simulink model "Model"  (R2023b)
settings: Solver=FixedStepAuto  StartTime=0.0  StopTime=10  FixedStep=0.002  RelTol=1e-3
model workspace (MAT data in the model file):
  a = 0
undefined symbols (not defined in the file or in its folder): X, Y, Z
libraries: sm_lib x84, nesl_utility x29, slpidlib x9, simulink x6
(part 4 of 7)

== matlab function Model/支持力结算/MATLAB Function3 ==
  data: m_w input; F_N output; T1 input; T2 input; a_w input; theta input; phi_1 input; phi_4 input; L_0 input
function F_N = fcn(m_w,T1,T2,a_w,theta,phi_1,phi_4,L_0)

l_1=0.15;
l_2=0.27;
l_3=0.27;
l_4=0.15;
l_5=0.15;g=9.80665;

J11=(2*(l_1*cos(phi_1) + (2*l_2*cos(2*atan(((4*l_2^2*(l_1*sin(phi_1) - l_4*sin(phi_4))^2 - ((l_1*sin(phi_1) - l_4*sin(phi_4))^2 + (l_5 - l_1*cos(phi_1) + l_4*cos(phi_4))^2 + l_2^2 - l_3^2)^2 + 4*l_2^2*(l_5 - l_1*cos(phi_1) + l_4*cos(phi_4))^2)^(1/2) - 2*l_2*(l_1*sin(phi_1) - l_4*sin(phi_4)))/((l_1*sin(phi_1) - l_4*sin(phi_4))^2 + (l_5 - l_1*cos(phi_1) + l_4*cos(phi_4))^2 + l_2^2 - l_3^2 + 2*l_2*(l_5 - l_1*cos(phi_1) + l_4*cos(phi_4)))))*(((8*l_1*l_2^2*cos(phi_1)*(l_1*sin(phi_1) - l_4*sin(phi_4)) - 2*(2*l_1*cos(phi_1)*(l_1*sin(phi_1) - l_4*sin(phi_4)) + 2*l_1*sin(phi_1)*(l_5 - l_1*cos(phi_1) + l_4*cos(phi_4)))*((l_1*sin(phi_1) - l_4*sin(phi_4))^2 + (l_5 - l_1*cos(phi_1) + l_4*cos(phi_4))^2 + l_2^2 - l_3^2) + 8*l_1*l_2^2*sin(phi_1)*(l_5 - l_1*cos(phi_1) + l_4*cos(phi_4)))/(2*(4*l_2^2*(l_1*sin(phi_1) - l_4*sin(phi_4))^2 - ((l_1*sin(phi_1) - l_4*sin(phi_4))^2 + (l_5 - l_1*cos(phi_1) + l_4*cos(phi_4))^2 + l_2^2 - l_3^2)^2 + 4*l_2^2*(l_5 - l_1*cos(phi_1) + l_4*cos(phi_4))^2)^(1/2)) - 2*l_1*l_2*cos(phi_1))/((l_1*sin(phi_1) - l_4*sin(phi_4))^2 + (l_5 - l_1*cos(phi_1) + l_4*cos(phi_4))^2 + l_2^2 - l_3^2 + 2*l_2*(l_5 - l_1*cos(phi_1) + l_4*cos(phi_4))) - (((4*l_2^2*(l_1*sin(phi_1) - l_4*sin(phi_4))^2 - ((l_1*sin(phi_1) - l_4*sin(phi_4))^2 + (l_5 - l_1*cos(phi_1) + l_4*cos(phi_4))^2 + l_2^2 - l_3^2)^2 + 4*l_2^2*(l_5 - l_1*cos(phi_1) + l_4*cos(phi_4))^2)^(1/2) - 2*l_2*(l_1*sin(phi_1) - l_4*sin(phi_4)))*(2*l_1*l_2*sin(phi_1) + 2*l_1*cos(phi_1)*(l_1*sin(phi_1) - l_4*sin(phi_4)) + 2*l_1*sin(phi_1)*(l_5 - l_1*cos(phi_1) + l_4*cos(phi_4))))/((l_1*sin(phi_1) - l_4*sin(phi_4))^2 + (l_5 - l_1*cos(phi_1) + l_4*cos(phi_4))^2 + l_2^2 - l_3^2 + 2*l_2*(l_5 - l_1*cos(phi_1) + l_4*cos(phi_4)))^2))/(((4*l_2^2*(l_1*sin(phi_1) - l_4*sin(phi_4))^2 - ((l_1*sin(phi_1) - l_4*sin(phi_4))^2 + (l_5 - l_1*cos(phi_1) + l_4*cos(phi_4))^2 + l_2^2 - l_3^2)^2 + 4*l_2^2*(l_5 - l_1*cos(phi_1) + l_4*cos(phi_4))^2)^(1/2) - 2*l_2*(l_1*sin(phi_1) - l_4*sin(phi_4)))^2/((l_1*sin(phi_1) - l_4*sin(phi_4))^2 + (l_5 - l_1*cos(phi_1) + l_4*cos(phi_4))^2 + l_2^2 - l_3^2 + 2*l_2*(l_5 - l_1*cos(phi_1) + l_4*cos(phi_4)))^2 + 1))*(l_2*sin(2*atan(((4*l_2^2*(l_1*sin(phi_1) - l_4*sin(phi_4))^2 - ((l_1*sin(phi_1) - l_4*sin(phi_4))^2 + (l_5 - l_1*cos(phi_1) + l_4*cos(phi_4))^2 + l_2^2 - l_3^2)^2 + 4*l_2^2*(l_5 - l_1*cos(phi_1) + l_4*cos(phi_4))^2)^(1/2) - 2*l_2*(l_1*sin(phi_1) - l_4*sin(phi_4)))/((l_1*sin(phi_1) - l_4*sin(phi_4))^2 + (l_5 - l_1*cos(phi_1) + l_4*cos(phi_4))^2 + l_2^2 - l_3^2 + 2*l_2*(l_5 - l_1*cos(phi_1) + l_4*cos(phi_4))))) + l_1*sin(phi_1)) - 2*(l_1*sin(phi_1) + (2*l_2*sin(2*atan(((4*l_2^2*(l_1*sin(phi_1) - l_4*sin(phi_4))^2 - ((l_1*sin(phi_1) - l_4*sin(phi_4))^2 + (l_5 - l_1*cos(phi_1) + l_4*cos(phi_4))^2 + l_2^2 - l_3^2)^2 + 4*l_2^2*(l_5 - l_1*cos(phi_1) + l_4*cos(phi_4))^2)^(1/2) - 2*l_2*(l_1*sin(phi_1) - l_4*sin(phi_4)))/((l_1*sin(phi_1) - l_4*sin(phi_4))^2 + (l_5 - l_1*cos(phi_1) + l_4*cos(phi_4))^2 + l_2^2 - l_3^2 + 2*l_2*(l_5 - l_1*cos(phi_1) + l_4*cos(phi_4)))))*(((8*l_1*l_2^2*cos(phi_1)*(l_1*sin(phi_1) - l_4*sin(phi_4)) - 2*(2*l_1*cos(phi_1)*(l_1*sin(phi_1) - l_4*sin(phi_4)) + 2*l_1*sin(phi_1)*(l_5 - l_1*cos(phi_1) + l_4*cos(phi_4)))*((l_1*sin(phi_1) - l_4*sin(phi_4))^2 + (l_5 - l_1*cos(phi_1) + l_4*cos(phi_4))^2 + l_2^2 - l_3^2) + 8*l_1*l_2^2*sin(phi_1)*(l_5 - l_1*cos(phi_1) + l_4*cos(phi_4)))/(2*(4*l_2^2*(l_1*sin(phi_1) - l_4*sin(phi_4))^2 - ((l_1*sin(phi_1) - l_4*sin(phi_4))^2 + (l_5 - l_1*cos(phi_1) + l_4*cos(phi_4))^2 + l_2^2 - l_3^2)^2 + 4*l_2^2*(l_5 - l_1*cos(phi_1) + l_4*cos(phi_4))^2)^(1/2)) - 2*l_1*l_2*cos(phi_1))/((l_1*sin(phi_1) - l_4*sin(phi_4))^2 + (l_5 - l_1*cos(phi_1) + l_4*cos(phi_4))^2 + l_2^2 - l_3^2 + 2*l_2*(l_5 - l_1*cos(phi_1) + l_4*cos(phi_4))) - (((4*l_2^2*(l_1*sin(phi_1) - l_4*sin(phi_4))^2 - ((l_1*sin(phi_1) - l_4*sin(phi_4))^2 + (l_5 - l_1*cos(phi_1) + l_4*cos(phi_4))^2 + l_2^2 - l_3^2)^2 + 4*l_2^2*(l_5 - l_1*cos(phi_1) + l_4*cos(phi_4))^2)^(1/2) - 2*l_2*(l_1*sin(phi_1) - l_4*sin(phi_4)))*(2*l_1*l_2*sin(phi_1) + 2*l_1*cos(phi_1)*(l_1*sin(phi_1) - l_4*sin(phi_4)) + 2*l_1*sin(phi_1)*(l_5 - l_1*cos(phi_1) + l_4*cos(phi_4))))/((l_1*sin(phi_1) - l_4*sin(phi_4))^2 + (l_5 - l_1*cos(phi_1) + l_4*cos(phi_4))^2 + l_2^2 - l_3^2 + 2*l_2*(l_5 - l_1*cos(phi_1) + l_4*cos(phi_4)))^2))/(((4*l_2^2*(l_1*sin(phi_1) - l_4*sin(phi_4))^2 - ((l_1*sin(phi_1) - l_4*sin(phi_4))^2 + (l_5 - l_1*cos(phi_1) + l_4*cos(phi_4))^2 + l_2^2 - l_3^2)^2 + 4*l_2^2*(l_5 - l_1*cos(phi_1) + l_4*cos(phi_4))^2)^(1/2) - 2*l_2*(l_1*sin(phi_1) - l_4*sin(phi_4)))^2/((l_1*sin(phi_1) - l_4*sin(phi_4))^2 + (l_5 - l_1*cos(phi_1) + l_4*cos(phi_4))^2 + l_2^2 - l_3^2 + 2*l_2*(l_5 - l_1*cos(phi_1) + l_4*cos(phi_4)))^2 + 1))*(l_2*cos(2*atan(((4*l_2^2*(l_1*sin(phi_1) - l_4*sin(phi_4))^2 - ((l_1*sin(phi_1) - l_4*sin(phi_4))^2 + (l_5 - l_1*cos(phi_1) + l_4*cos(phi_4))^2 + l_2^2 - l_3^2)^2 + 4*l_2^2*(l_5 - l_1*cos(phi_1) + l_4*cos(phi_4))^2)^(1/2) - 2*l_2*(l_1*sin(phi_1) - l_4*sin(phi_4)))/((l_1*sin(phi_1) - l_4*sin(phi_4))^2 + (l_5 - l_1*cos(phi_1) + l_4*cos(phi_4))^2 + l_2^2 - l_3^2 + 2*l_2*(l_5 - l_1*cos(phi_1) + l_4*cos(phi_4))))) - l_5/2 + l_1*cos(phi_1)))/(2*((l_2*sin(2*atan(((4*l_2^2*(l_1*sin(phi_1) - l_4*sin(phi_4))^2 - ((l_1*sin(phi_1) - l_4*sin(phi_4))^2 + (l_5 - l_1*cos(phi_1) + l_4*cos(phi_4))^2 + l_2^2 - l_3^2)^2 + 4*l_2^2*(l_5 - l_1*cos(phi_1) + l_4*cos(phi_4))^2)^(1/2) - 2*l_2*(l_1*sin(phi_1) - l_4*sin(phi_4)))/((l_1*sin(phi_1) - l_4*sin(phi_4))^2 + (l_5 - l_1*cos(phi_1) + l_4*cos(phi_4))^2 + l_2^2 - l_3^2 + 2*l_2*(l_5 - l_1*cos(phi_1) + l_4*cos(phi_4))))) + l_1*sin(phi_1))^2 + (l_2*cos(2*atan(((4*l_2^2*(l_1*sin(phi_1) - l_4*sin(phi_4))^2 - ((l_1*sin(phi_1) - l_4*sin(phi_4))^2 + (l_5 - l_1*cos(phi_1) + l_4*cos(phi_4))^2 + l_2^2 - l_3^2)^2 + 4*l_2^2*(l_5 - l_1*cos(phi_1) + l_4*cos(phi_4))^2)^(1/2) - 2*l_2*(l_1*sin(phi_1) - l_4*sin(phi_4)))/((l_1*sin(phi_1) - l_4*sin(phi_4))^2 + (l_5 - l_1*cos(phi_1) + l_4*cos(phi_4))^2 + l_2^2 - l_3^2 + 2*l_2*(l_5 - l_1*cos(phi_1) + l_4*cos(phi_4))))) - l_5/2 + l_1*cos(phi_1))^2)^(1/2));
J12=((4*l_2*sin(2*atan(((4*l_2^2*(l_1*sin(phi_1) - l_4*sin(phi_4))^2 - ((l_1*sin(phi_1) - l_4*sin(phi_4))^2 + (l_5 - l_1*cos(phi_1) + l_4*cos(phi_4))^2 + l_2^2 - l_3^2)^2 + 4*l_2^2*(l_5 - l_1*cos(phi_1) + l_4*cos(phi_4))^2)^(1/2) - 2*l_2*(l_1*sin(phi_1) - l_4*sin(phi_4)))/((l_1*sin(phi_1) - l_4*sin(phi_4))^2 + (l_5 - l_1*cos(phi_1) + l_4*cos(phi_4))^2 + l_2^2 - l_3^2 + 2*l_2*(l_5 - l_1*cos(phi_1) + l_4*cos(phi_4)))))*(((8*l_2^2*l_4*cos(phi_4)*(l_1*sin(phi_1) - l_4*sin(phi_4)) - 2*(2*l_4*cos(phi_4)*(l_1*sin(phi_1) - l_4*sin(phi_4)) + 2*l_4*sin(phi_4)*(l_5 - l_1*cos(phi_1) + l_4*cos(phi_4)))*((l_1*sin(phi_1) - l_4*sin(phi_4))^2 + (l_5 - l_1*cos(phi_1) + l_4*cos(phi_4))^2 + l_2^2 - l_3^2) + 8*l_2^2*l_4*sin(phi_4)*(l_5 - l_1*cos(phi_1) + l_4*cos(phi_4)))/(2*(4*l_2^2*(l_1*sin(phi_1) - l_4*sin(phi_4))^2 - ((l_1*sin(phi_1) - l_4*sin(phi_4))^2 + (l_5 - l_1*cos(phi_1) + l_4*cos(phi_4))^2 + l_2^2 - l_3^2)^2 + 4*l_2^2*(l_5 - l_1*cos(phi_1) + l_4*cos(phi_4))^2)^(1/2)) - 2*l_2*l_4*cos(phi_4))/((l_1*sin(phi_1) - l_4*sin(phi_4))^2 + (l_5 - l_1*cos(phi_1) + l_4*cos(phi_4))^2 + l_2^2 - l_3^2 + 2*l_2*(l_5 - l_1*cos(phi_1) + l_4*cos(phi_4))) - (((4*l_2^2*(l_1*sin(phi_1) - l_4*sin(phi_4))^2 - ((l_1*sin(phi_1) - l_4*sin(phi_4))^2 + (l_5 - l_1*cos(phi_1) + l_4*cos(phi_4))^2 + l_2^2 - l_3^2)^2 + 4*l_2^2*(l_5 - l_1*cos(phi_1) + l_4*cos(phi_4))^2)^(1/2) - 2*l_2*(l_1*sin(phi_1) - l_4*sin(phi_4)))*(2*l_2*l_4*sin(phi_4) + 2*l_4*cos(phi_4)*(l_1*sin(phi_1) - l_4*sin(phi_4)) + 2*l_4*sin(phi_4)*(l_5 - l_1*cos(phi_1) + l_4*cos(phi_4))))/((l_1*sin(phi_1) - l_4*sin(phi_4))^2 + (l_5 - l_1*cos(phi_1) + l_4*cos(phi_4))^2 + l_2^2 - l_3^2 + 2*l_2*(l_5 - l_1*cos(phi_1) + l_4*cos(phi_4)))^2)*(l_2*cos(2*atan(((4*l_2^2*(l_1*sin(phi_1) - l_4*sin(phi_4))^2 - ((l_1*sin(phi_1) - l_4*sin(phi_4))^2 + (l_5 - l_1*cos(phi_1) + l_4*cos(phi_4))^2 + l_2^2 - l_3^2)^2 + 4*l_2^2*(l_5 - l_1*cos(phi_1) + l_4*cos(phi_4))^2)^(1/2) - 2*l_2*(l_1*sin(phi_1) - l_4*sin(phi_4)))/((l_1*sin(phi_1) - l_4*sin(phi_4))^2 + (l_5 - l_1*cos(phi_1) + l_4*cos(phi_4))^2 + l_2^2 - l_3^2 + 2*l_2*(l_5 - l_1*cos(phi_1) + l_4*cos(phi_4))))) - l_5/2 + l_1*cos(phi_1)))/(((4*l_2^2*(l_1*sin(phi_1) - l_4*sin(phi_4))^2 - ((l_1*sin(phi_1) - l_4*sin(phi_4))^2 + (l_5 - l_1*cos(phi_1) + l_4*cos(phi_4))^2 + l_2^2 - l_3^2)^2 + 4*l_2^2*(l_5 - l_1*cos(phi_1) + l_4*cos(phi_4))^2)^(1/2) - 2*l_2*(l_1*sin(phi_1) - l_4*sin(phi_4)))^2/((l_1*sin(phi_1) - l_4*sin(phi_4))^2 + (l_5 - l_1*cos(phi_1) + l_4*cos(phi_4))^2 + l_2^2 - l_3^2 + 2*l_2*(l_5 - l_1*cos(phi_1) + l_4*cos(phi_4)))^2 + 1) - (4*l_2*cos(2*atan(((4*l_2^2*(l_1*sin(phi_1) - l_4*sin(phi_4))^2 - ((l_1*sin(phi_1) - l_4*sin(phi_4))^2 + (l_5 - l_1*cos(phi_1) + l_4*cos(phi_4))^2 + l_2^2 - l_3^2)^2 + 4*l_2^2*(l_5 - l_1*cos(phi_1) + l_4*cos(phi_4))^2)^(1/2) - 2*l_2*(l_1*sin(phi_1) - l_4*sin(phi_4)))/((l_1*sin(phi_1) - l_4*sin(phi_4))^2 + (l_5 - l_1*cos(phi_1) + l_4*cos(phi_4))^2 + l_2^2 - l_3^2 + 2*l_2*(l_5 - l_1*cos(phi_1) + l_4*cos(phi_4)))))*(l_2*sin(2*atan(((4*l_2^2*(l_1*sin(phi_1) - l_4*sin(phi_4))^2 - ((l_1*sin(phi_1) - l_4*sin(phi_4))^2 + (l_5 - l_1*cos(phi_1) + l_4*cos(phi_4))^2 + l_2^2 - l_3^2)^2 + 4*l_2^2*(l_5 - l_1*cos(phi_1) + l_4*cos(phi_4))^2)^(1/2) - 2*l_2*(l_1*sin(phi_1) - l_4*sin(phi_4)))/((l_1*sin(phi_1) - l_4*sin(phi_4))^2 + (l_5 - l_1*cos(phi_1) + l_4*cos(phi_4))^2 + l_2^2 - l_3^2 + 2*l_2*(l_5 - l_1*cos(phi_1) + l_4*cos(phi_4))))) + l_1*sin(phi_1))*(((8*l_2^2*l_4*cos(phi_4)*(l_1*sin(phi_1) - l_4*sin(phi_4)) - 2*(2*l_4*cos(phi_4)*(l_1*sin(phi_1) - l_4*sin(phi_4)) + 2*l_4*sin(phi_4)*(l_5 - l_1*cos(phi_1) + l_4*cos(phi_4)))*((l_1*sin(phi_1) - l_4*sin(phi_4))^2 + (l_5 - l_1*cos(phi_1) + l_4*cos(phi_4))^2 + l_2^2 - l_3^2) + 8*l_2^2*l_4*sin(phi_4)*(l_5 - l_1*cos(phi_1) + l_4*cos(phi_4)))/(2*(4*l_2^2*(l_1*sin(phi_1) - l_4*sin(phi_4))^2 - ((l_1*sin(phi_1) - l_4*sin(phi_4))^2 + (l_5 - l_1*cos(phi_1) + l_4*cos(phi_4))^2 + l_2^2 - l_3^2)^2 + 4*l_2^2*(l_5 - l_1*cos(phi_1) + l_4*cos(phi_4))^2)^(1/2)) - 2*l_2*l_4*cos(phi_4))/((l_1*sin(phi_1) - l_4*sin(phi_4))^2 + (l_5 - l_1*cos(phi_1) + l_4*cos(phi_4))^2 + l_2^2 - l_3^2 + 2*l_2*(l_5 - l_1*cos(phi_1) + l_4*cos(phi_4))) - (((4*l_2^2*(l_1*sin(phi_1) - l_4*sin(phi_4))^2 - ((l_1*sin(phi_1) - l_4*sin(phi_4))^2 + (l_5 - l_1*cos(phi_1) + l_4*cos(phi_4))^2 + l_2^2 - l_3^2)^2 + 4*l_2^2*(l_5 - l_1*cos(phi_1) + l_4*cos(phi_4))^2)^(1/2) - 2*l_2*(l_1*sin(phi_1) - l_4*sin(phi_4)))*(2*l_2*l_4*sin(phi_4) + 2*l_4*cos(phi_4)*(l_1*sin(phi_1) - l_4*sin(phi_4)) + 2*l_4*sin(phi_4)*(l_5 - l_1*cos(phi_1) + l_4*cos(phi_4))))/((l_1*sin(phi_1) - l_4*sin(phi_4))^2 + (l_5 - l_1*cos(phi_1) + l_4*cos(phi_4))^2 + l_2^2 - l_3^2 + 2*l_2*(l_5 - l_1*cos(phi_1) + l_4*cos(phi_4)))^2))/(((4*l_2^2*(l_1*sin(phi_1) - l_4*sin(phi_4))^2 - ((l_1*sin(phi_1) - l_4*sin(phi_4))^2 + (l_5 - l_1*cos(phi_1) + l_4*cos(phi_4))^2 + l_2^2 - l_3^2)^2 + 4*l_2^2*(l_5 - l_1*cos(phi_1) + l_4*cos(phi_4))^2)^(1/2) - 2*l_2*(l_1*sin(phi_1) - l_4*sin(phi_4)))^2/((l_1*sin(phi_1) - l_4*sin(phi_4))^2 + (l_5 - l_1*cos(phi_1) + l_4*cos(phi_4))^2 + l_2^2 - l_3^2 + 2*l_2*(l_5 - l_1*cos(phi_1) + l_4*cos(phi_4)))^2 + 1))/(2*((l_2*sin(2*atan(((4*l_2^2*(l_1*sin(phi_1) - l_4*sin(phi_4))^2 - ((l_1*sin(phi_1) - l_4*sin(phi_4))^2 + (l_5 - l_1*cos(phi_1) + l_4*cos(phi_4))^2 + l_2^2 - l_3^2)^2 + 4*l_2^2*(l_5 - l_1*cos(phi_1) + l_4*cos(phi_4))^2)^(1/2) - 2*l_2*(l_1*sin(phi_1) - l_4*sin(phi_4)))/((l_1*sin(phi_1) - l_4*sin(phi_4))^2 + (l_5 - l_1*cos(phi_1) + l_4*cos(phi_4))^2 + l_2^2 - l_3^2 + 2*l_2*(l_5 - l_1*cos(phi_1) + l_4*cos(phi_4))))) + l_1*sin(phi_1))^2 + (l_2*cos(2*atan(((4*l_2^2*(l_1*sin(phi_1) - l_4*sin(phi_4))^2 - ((l_1*sin(phi_1) - l_4*sin(phi_4))^2 + (l_5 - l_1*cos(phi_1) + l_4*cos(phi_4))^2 + l_2^2 - l_3^2)^2 + 4*l_2^2*(l_5 - l_1*cos(phi_1) + l_4*cos(phi_4))^2)^(1/2) - 2*l_2*(l_1*sin(phi_1) - l_4*sin(phi_4)))/((l_1*sin(phi_1) - l_4*sin(phi_4))^2 + (l_5 - l_1*cos(phi_1) + l_4*cos(phi_4))^2 + l_2^2 - l_3^2 + 2*l_2*(l_5 - l_1*cos(phi_1) + l_4*cos(phi_4))))) - l_5/2 + l_1*cos(phi_1))^2)^(1/2));
J21=((l_1*sin(phi_1) + (2*l_2*sin(2*atan(((4*l_2^2*(l_1*sin(phi_1) - l_4*sin(phi_4))^2 - ((l_1*sin(phi_1) - l_4*sin(phi_4))^2 + (l_5 - l_1*cos(phi_1) + l_4*cos(phi_4))^2 + l_2^2 - l_3^2)^2 + 4*l_2^2*(l_5 - l_1*cos(phi_1) + l_4*cos(phi_4))^2)^(1/2) - 2*l_2*(l_1*sin(phi_1) - l_4*sin(phi_4)))/((l_1*sin(phi_1) - l_4*sin(phi_4))^2 + (l_5 - l_1*cos(phi_1) + l_4*cos(phi_4))^2 + l_2^2 - l_3^2 + 2*l_2*(l_5 - l_1*cos(phi_1) + l_4*cos(phi_4)))))*(((8*l_1*l_2^2*cos(phi_1)*(l_1*sin(phi_1) - l_4*sin(phi_4)) - 2*(2*l_1*cos(phi_1)*(l_1*sin(phi_1) - l_4*sin(phi_4)) + 2*l_1*sin(phi_1)*(l_5 - l_1*cos(phi_1) + l_4*cos(phi_4)))*((l_1*sin(phi_1) - l_4*sin(phi_4))^2 + (l_5 - l_1*cos(phi_1) + l_4*cos(phi_4))^2 + l_2^2 - l_3^2) + 8*l_1*l_2^2*sin(phi_1)*(l_5 - l_1*cos(phi_1) + l_4*cos(phi_4)))/(2*(4*l_2^2*(l_1*sin(phi_1) - l_4*sin(phi_4))^2 - ((l_1*sin(phi_1) - l_4*sin(phi_4))^2 + (l_5 - l_1*cos(phi_1) + l_4*cos(phi_4))^2 + l_2^2 - l_3^2)^2 + 4*l_2^2*(l_5 - l_1*cos(phi_1) + l_4*cos(phi_4))^2)^(1/2)) - 2*l_1*l_2*cos(phi_1))/((l_1*sin(phi_1) - l_4*sin(phi_4))^2 + (l_5 - l_1*cos(phi_1) + l_4*cos(phi_4))^2 + l_2^2 - l_3^2 + 2*l_2*(l_5 - l_1*cos(phi_1) + l_4*cos(phi_4))) - (((4*l_2^2*(l_1*sin(phi_1) - l_4*sin(phi_4))^2 - ((l_1*sin(phi_1) - l_4*sin(phi_4))^2 + (l_5 - l_1*cos(phi_1) + l_4*cos(phi_4))^2 + l_2^2 - l_3^2)^2 + 4*l_2^2*(l_5 - l_1*cos(phi_1) + l_4*cos(phi_4))^2)^(1/2) - 2*l_2*(l_1*sin(phi_1) - l_4*sin(phi_4)))*(2*l_1*l_2*sin(phi_1) + 2*l_1*cos(phi_1)*(l_1*sin(phi_1) - l_4*sin(phi_4)) + 2*l_1*sin(phi_1)*(l_5 - l_1*cos(phi_1) + l_4*cos(phi_4))))/((l_1*sin(phi_1) - l_4*sin(phi_4))^2 + (l_5 - l_1*cos(phi_1) + l_4*cos(phi_4))^2 + l_2^2 - l_3^2 + 2*l_2*(l_5 - l_1*cos(phi_1) + l_4*cos(phi_4)))^2))/(((4*l_2^2*(l_1*sin(phi_1) - l_4*sin(phi_4))^2 - ((l_1*sin(phi_1) - l_4*sin(phi_4))^2 + (l_5 - l_1*cos(phi_1) + l_4*cos(phi_4))^2 + l_2^2 - l_3^2)^2 + 4*l_2^2*(l_5 - l_1*cos(phi_1) + l_4*cos(phi_4))^2)^(1/2) - 2*l_2*(l_1*sin(phi_1) - l_4*sin(phi_4)))^2/((l_1*sin(phi_1) - l_4*sin(phi_4))^2 + (l_5 - l_1*cos(phi_1) + l_4*cos(phi_4))^2 + l_2^2 - l_3^2 + 2*l_2*(l_5 - l_1*cos(phi_1) + l_4*cos(phi_4)))^2 + 1))/((l_2*sin(2*atan(((4*l_2^2*(l_1*sin(phi_1) - l_4*sin(phi_4))^2 - ((l_1*sin(phi_1) - l_4*sin(phi_4))^2 + (l_5 - l_1*cos(phi_1) + l_4*cos(phi_4))^2 + l_2^2 - l_3^2)^2 + 4*l_2^2*(l_5 - l_1*cos(phi_1) + l_4*cos(phi_4))^2)^(1/2) - 2*l_2*(l_1*sin(phi_1) - l_4*sin(phi_4)))/((l_1*sin(phi_1) - l_4*sin(phi_4))^2 + (l_5 - l_1*cos(phi_1) + l_4*cos(phi_4))^2 + l_2^2 - l_3^2 + 2*l_2*(l_5 - l_1*cos(phi_1) + l_4*cos(phi_4))))) + l_1*sin(phi_1))^2 + (l_2*cos(2*atan(((4*l_2^2*(l_1*sin(phi_1) - l_4*sin(phi_4))^2 - ((l_1*sin(phi_1) - l_4*sin(phi_4))^2 + (l_5 - l_1*cos(phi_1) + l_4*cos(phi_4))^2 + l_2^2 - l_3^2)^2 + 4*l_2^2*(l_5 - l_1*cos(phi_1) + l_4*cos(phi_4))^2)^(1/2) - 2*l_2*(l_1*sin(phi_1) - l_4*sin(phi_4)))/((l_1*sin(phi_1) - l_4*sin(phi_4))^2 + (l_5 - l_1*cos(phi_1) + l_4*cos(phi_4))^2 + l_2^2 - l_3^2 + 2*l_2*(l_5 - l_1*cos(phi_1) + l_4*cos(phi_4))))) - l_5/2 + l_1*cos(phi_1))^2)^(1/2) + ((2*(l_1*cos(phi_1) + (2*l_2*cos(2*atan(((4*l_2^2*(l_1*sin(phi_1) - l_4*sin(phi_4))^2 - ((l_1*sin(phi_1) - l_4*sin(phi_4))^2 + (l_5 - l_1*cos(phi_1) + l_4*cos(phi_4))^2 + l_2^2 - l_3^2)^2 + 4*l_2^2*(l_5 - l_1*cos(phi_1) + l_4*cos(phi_4))^2)^(1/2) - 2*l_2*(l_1*sin(phi_1) - l_4*sin(phi_4)))/((l_1*sin(phi_1) - l_4*sin(phi_4))^2 + (l_5 - l_1*cos(phi_1) + l_4*cos(phi_4))^2 + l_2^2 - l_3^2 + 2*l_2*(l_5 - l_1*cos(phi_1) + l_4*cos(phi_4)))))*(((8*l_1*l_2^2*cos(phi_1)*(l_1*sin(phi_1) - l_4*sin(phi_4)) - 2*(2*l_1*cos(phi_1)*(l_1*sin(phi_1) - l_4*sin(phi_4)) + 2*l_1*sin(phi_1)*(l_5 - l_1*cos(phi_1) + l_4*cos(phi_4)))*((l_1*sin(phi_1) - l_4*sin(phi_4))^2 + (l_5 - l_1*cos(phi_1) + l_4*cos(phi_4))^2 + l_2^2 - l_3^2) + 8*l_1*l_2^2*sin(phi_1)*(l_5 - l_1*cos(phi_1) + l_4*cos(phi_4)))/(2*(4*l_2^2*(l_1*sin(phi_1) - l_4*sin(phi_4))^2 - ((l_1*sin(phi_1) - l_4*sin(phi_4))^2 + (l_5 - l_1*cos(phi_1) + l_4*cos(phi_4))^2 + l_2^2 - l_3^2)^2 + 4*l_2^2*(l_5 - l_1*cos(phi_1) + l_4*cos(phi_4))^2)^(1/2)) - 2*l_1*l_2*cos(phi_1))/((l_1*sin(phi_1) - l_4*sin(phi_4))^2 + (l_5 - l_1*cos(phi_1) + l_4*cos(phi_4))^2 + l_2^2 - l_3^2 + 2*l_2*(l_5 - l_1*cos(phi_1) + l_4*cos(phi_4))) - (((4*l_2^2*(l_1*sin(phi_1) - l_4*sin(phi_4))^2 - ((l_1*sin(phi_1) - l_4*sin(phi_4))^2 + (l_5 - l_1*cos(phi_1) + l_4*cos(phi_4))^2 + l_2^2 - l_3^2)^2 + 4*l_2^2*(l_5 - l_1*cos(phi_1) + l_4*cos(phi_4))^2)^(1/2) - 2*l_2*(l_1*sin(phi_1) - l_4*sin(phi_4)))*(2*l_1*l_2*sin(phi_1) + 2*l_1*cos(phi_1)*(l_1*sin(phi_1) - l_4*sin(phi_4)) + 2*l_1*sin(phi_1)*(l_5 - l_1*cos(phi_1) + l_4*cos(phi_4))))/((l_1*sin(phi_1) - l_4*sin(phi_4))^2 + (l_5 - l_1*cos(phi_1) + l_4*cos(phi_4))^2 + l_2^2 - l_3^2 + 2*l_2*(l_5 - l_1*cos(phi_1) + l_4*cos(phi_4)))^2))/(((4*l_2^2*(l_1*sin(phi_1) - l_4*sin(phi_4))^2 - ((l_1*sin(phi_1) - l_4*sin(phi_4))^2 + (l_5 - l_1*cos(phi_1) + l_4*cos(phi_4))^2 + l_2^2 - l_3^2)^2 + 4*l_2^2*(l_5 - l_1*cos(phi_1) + l_4*cos(phi_4))^2)^(1/2) - 2*l_2*(l_1*sin(phi_1) - l_4*sin(phi_4)))^2/((l_1*sin(phi_1) - l_4*sin(phi_4))^2 + (l_5 - l_1*cos(phi_1) + l_4*cos(phi_4))^2 + l_2^2 - l_3^2 + 2*l_2*(l_5 - l_1*cos(phi_1) + l_4*cos(phi_4)))^2 + 1))*(l_2*sin(2*atan(((4*l_2^2*(l_1*sin(phi_1) - l_4*sin(phi_4))^2 - ((l_1*sin(phi_1) - l_4*sin(phi_4))^2 + (l_5 - l_1*cos(phi_1) + l_4*cos(phi_4))^2 + l_2^2 - l_3^2)^2 + 4*l_2^2*(l_5 - l_1*cos(phi_1) + l_4*cos(phi_4))^2)^(1/2) - 2*l_2*(l_1*sin(phi_1) - l_4*sin(phi_4)))/((l_1*sin(phi_1) - l_4*sin(phi_4))^2 + (l_5 - l_1*cos(phi_1) + l_4*cos(phi_4))^2 + l_2^2 - l_3^2 + 2*l_2*(l_5 - l_1*cos(phi_1) + l_4*cos(phi_4))))) + l_1*sin(phi_1)) - 2*(l_1*sin(phi_1) + (2*l_2*sin(2*atan(((4*l_2^2*(l_1*sin(phi_1) - l_4*sin(phi_4))^2 - ((l_1*sin(phi_1) - l_4*sin(phi_4))^2 + (l_5 - l_1*cos(phi_1) + l_4*cos(phi_4))^2 + l_2^2 - l_3^2)^2 + 4*l_2^2*(l_5 - l_1*cos(phi_1) + l_4*cos(phi_4))^2)^(1/2) - 2*l_2*(l_1*sin(phi_1) - l_4*sin(phi_4)))/((l_1*sin(phi_1) - l_4*sin(phi_4))^2 + (l_5 - l_1*cos(phi_1) + l_4*cos(phi_4))^2 + l_2^2 - l_3^2 + 2*l_2*(l_5 - l_1*cos(phi_1) + l_4*cos(phi_4)))))*(((8*l_1*l_2^2*cos(phi_1)*(l_1*sin(phi_1) - l_4*sin(phi_4)) - 2*(2*l_1*cos(phi_1)*(l_1*sin(phi_1) - l_4*sin(phi_4)) + 2*l_1*sin(phi_1)*(l_5 - l_1*cos(phi_1) + l_4*cos(phi_4)))*((l_1*sin(phi_1) - l_4*sin(phi_4))^2 + (l_5 - l_1*cos(phi_1) + l_4*cos(phi_4))^2 + l_2^2 - l_3^2) + 8*l_1*l_2^2*sin(phi_1)*(l_5 - l_1*cos(phi_1) + l_4*cos(phi_4)))/(2*(4*l_2^2*(l_1*sin(phi_1) - l_4*sin(phi_4))^2 - ((l_1*sin(phi_1) - l_4*sin(phi_4))^2 + (l_5 - l_1*cos(phi_1) + l_4*cos(phi_4))^2 + l_2^2 - l_3^2)^2 + 4*l_2^2*(l_5 - l_1*cos(phi_1) + l_4*cos(phi_4))^2)^(1/2)) - 2*l_1*l_2*cos(phi_1))/((l_1*sin(phi_1) - l_4*sin(phi_4))^2 + (l_5 - l_1*cos(phi_1) + l_4*cos(phi_4))^2 + l_2^2 - l_3^2 + 2*l_2*(l_5 - l_1*cos(phi_1) + l_4*cos(phi_4))) - (((4*l_2^2*(l_1*sin(phi_1) - l_4*sin(phi_4))^2 - ((l_1*sin(phi_1) - l_4*sin(phi_4))^2 + (l_5 - l_1*cos(phi_1) + l_4*cos(phi_4))^2 + l_2^2 - l_3^2)^2 + 4*l_2^2*(l_5 - l_1*cos(phi_1) + l_4*cos(phi_4))^2)^(1/2) - 2*l_2*(l_1*sin(phi_1) - l_4*sin(phi_4)))*(2*l_1*l_2*sin(phi_1) + 2*l_1*cos(phi_1)*(l_1*sin(phi_1) - l_4*sin(phi_4)) + 2*l_1*sin(phi_1)*(l_5 - l_1*cos(phi_1) + l_4*cos(phi_4))))/((l_1*sin(phi_1) - l_4*sin(phi_4))^2 + (l_5 - l_1*cos(phi_1) + l_4*cos(phi_4))^2 + l_2^2 - l_3^2 + 2*l_2*(l_5 - l_1*cos(phi_1) + l_4*cos(phi_4)))^2))/(((4*l_2^2*(l_1*sin(phi_1) - l_4*sin(phi_4))^2 - ((l_1*sin(phi_1) - l_4*sin(phi_4))^2 + (l_5 - l_1*cos(phi_1) + l_4*cos(phi_4))^2 + l_2^2 - l_3^2)^2 + 4*l_2^2*(l_5 - l_1*cos(phi_1) + l_4*cos(phi_4))^2)^(1/2) - 2*l_2*(l_1*sin(phi_1) - l_4*sin(phi_4)))^2/((l_1*sin(phi_1) - l_4*sin(phi_4))^2 + (l_5 - l_1*cos(phi_1) + l_4*cos(phi_4))^2 + l_2^2 - l_3^2 + 2*l_2*(l_5 - l_1*cos(phi_1) + l_4*cos(phi_4)))^2 + 1))*(l_2*cos(2*atan(((4*l_2^2*(l_1*sin(phi_1) - l_4*sin(phi_4))^2 - ((l_1*sin(phi_1) - l_4*sin(phi_4))^2 + (l_5 - l_1*cos(phi_1) + l_4*cos(phi_4))^2 + l_2^2 - l_3^2)^2 + 4*l_2^2*(l_5 - l_1*cos(phi_1) + l_4*cos(phi_4))^2)^(1/2) - 2*l_2*(l_1*sin(phi_1) - l_4*sin(phi_4)))/((l_1*sin(phi_1) - l_4*sin(phi_4))^2 + (l_5 - l_1*cos(phi_1) + l_4*cos(phi_4))^2 + l_2^2 - l_3^2 + 2*l_2*(l_5 - l_1*cos(phi_1) + l_4*cos(phi_4))))) - l_5/2 + l_1*cos(phi_1)))*(l_2*cos(2*atan(((4*l_2^2*(l_1*sin(phi_1) - l_4*sin(phi_4))^2 - ((l_1*sin(phi_1) - l_4*sin(phi_4))^2 + (l_5 - l_1*cos(phi_1) + l_4*cos(phi_4))^2 + l_2^2 - l_3^2)^2 + 4*l_2^2*(l_5 - l_1*cos(phi_1) + l_4*cos(phi_4))^2)^(1/2) - 2*l_2*(l_1*sin(phi_1) - l_4*sin(phi_4)))/((l_1*sin(phi_1) - l_4*sin(phi_4))^2 + (l_5 - l_1*cos(phi_1) + l_4*cos(phi_4))^2 + l_2^2 - l_3^2 + 2*l_2*(l_5 - l_1*cos(phi_1) + l_4*cos(phi_4))))) - l_5/2 + l_1*cos(phi_1)))/(2*((l_2*sin(2*atan(((4*l_2^2*(l_1*sin(phi_1) - l_4*sin(phi_4))^2 - ((l_1*sin(phi_1) - l_4*sin(phi_4))^2 + (l_5 - l_1*cos(phi_1) + l_4*cos(phi_4))^2 + l_2^2 - l_3^2)^2 + 4*l_2^2*(l_5 - l_1*cos(phi_1) + l_4*cos(phi_4))^2)^(1/2) - 2*l_2*(l_1*sin(phi_1) - l_4*sin(phi_4)))/((l_1*sin(phi_1) - l_4*sin(phi_4))^2 + (l_5 - l_1*cos(phi_1) + l_4*cos(phi_4))^2 + l_2^2 - l_3^2 + 2*l_2*(l_5 - l_1*cos(phi_1) + l_4*cos(phi_4))))) + l_1*sin(phi_1))^2 + (l_2*cos(2*atan(((4*l_2^2*(l_1*sin(phi_1) - l_4*sin(phi_4))^2 - ((l_1*sin(phi_1) - l_4*sin(phi_4))^2 + (l_5 - l_1*cos(phi_1) + l_4*cos(phi_4))^2 + l_2^2 - l_3^2)^2 + 4*l_2^2*(l_5 - l_1*cos(phi_1) + l_4*cos(phi_4))^2)^(1/2) - 2*l_2*(l_1*sin(phi_1) - l_4*sin(phi_4)))/((l_1*sin(phi_1) - l_4*sin(phi_4))^2 + (l_5 - l_1*cos(phi_1) + l_4*cos(phi_4))^2 + l_2^2 - l_3^2 + 2*l_2*(l_5 - l_1*cos(phi_1) + l_4*cos(phi_4))))) - l_5/2 + l_1*cos(phi_1))^2)^(3/2)))/(1 - (l_2*cos(2*atan(((4*l_2^2*(l_1*sin(phi_1) - l_4*sin(phi_4))^2 - ((l_1*sin(phi_1) - l_4*sin(phi_4))^2 + (l_5 - l_1*cos(phi_1) + l_4*cos(phi_4))^2 + l_2^2 - l_3^2)^2 + 4*l_2^2*(l_5 - l_1*cos(phi_1) + l_4*cos(phi_4))^2)^(1/2) - 2*l_2*(l_1*sin(phi_1) - l_4*sin(phi_4)))/((l_1*sin(phi_1) - l_4*sin(phi_4))^2 + (l_5 - l_1*cos(phi_1) + l_4*cos(phi_4))^2 + l_2^2 - l_3^2 + 2*l_2*(l_5 - l_1*cos(phi_1) + l_4*cos(phi_4))))) - l_5/2 + l_1*cos(phi_1))^2/((l_2*sin(2*atan(((4*l_2^2*(l_1*sin(phi_1) - l_4*sin(phi_4))^2 - ((l_1*sin(phi_1) - l_4*sin(phi_4))^2 + (l_5 - l_1*cos(phi_1) + l_4*cos(phi_4))^2 + l_2^2 - l_3^2)^2 + 4*l_2^2*(l_5 - l_1*cos(phi_1) + l_4*cos(phi_4))^2)^(1/2) - 2*l_2*(l_1*sin(phi_1) - l_4*sin(phi_4)))/((l_1*sin(phi_1) - l_4*sin(phi_4))^2 + (l_5 - l_1*cos(phi_1) + l_4*cos(phi_4))^2 + l_2^2 - l_3^2 + 2*l_2*(l_5 - l_1*cos(phi_1) + l_4*cos(phi_4))))) + l_1*sin(phi_1))^2 + (l_2*cos(2*atan(((4*l_2^2*(l_1*sin(phi_1) - l_4*sin(phi_4))^2 - ((l_1*sin(phi_1) - l_4*sin(phi_4))^2 + (l_5 - l_1*cos(phi_1) + l_4*cos(phi_4))^2 + l_2^2 - l_3^2)^2 + 4*l_2^2*(l_5 - l_1*cos(phi_1) + l_4*cos(phi_4))^2)^(1/2) - 2*l_2*(l_1*sin(phi_1) - l_4*sin(phi_4)))/((l_1*sin(phi_1) - l_4*sin(phi_4))^2 + (l_5 - l_1*cos(phi_1) + l_4*cos(phi_4))^2 + l_2^2 - l_3^2 + 2*l_2*(l_5 - l_1*cos(phi_1) + l_4*cos(phi_4))))) - l_5/2 + l_1*cos(phi_1))^2))^(1/2);
J22=((((4*l_2*sin(2*atan(((4*l_2^2*(l_1*sin(phi_1) - l_4*sin(phi_4))^2 - ((l_1*sin(phi_1) - l_4*sin(phi_4))^2 + (l_5 - l_1*cos(phi_1) + l_4*cos(phi_4))^2 + l_2^2 - l_3^2)^2 + 4*l_2^2*(l_5 - l_1*cos(phi_1) + l_4*cos(phi_4))^2)^(1/2) - 2*l_2*(l_1*sin(phi_1) - l_4*sin(phi_4)))/((l_1*sin(phi_1) - l_4*sin(phi_4))^2 + (l_5 - l_1*cos(phi_1) + l_4*cos(phi_4))^2 + l_2^2 - l_3^2 + 2*l_2*(l_5 - l_1*cos(phi_1) + l_4*cos(phi_4)))))*(((8*l_2^2*l_4*cos(phi_4)*(l_1*sin(phi_1) - l_4*sin(phi_4)) - 2*(2*l_4*cos(phi_4)*(l_1*sin(phi_1) - l_4*sin(phi_4)) + 2*l_4*sin(phi_4)*(l_5 - l_1*cos(phi_1) + l_4*cos(phi_4)))*((l_1*sin(phi_1) - l_4*sin(phi_4))^2 + (l_5 - l_1*cos(phi_1) + l_4*cos(phi_4))^2 + l_2^2 - l_3^2) + 8*l_2^2*l_4*sin(phi_4)*(l_5 - l_1*cos(phi_1) + l_4*cos(phi_4)))/(2*(4*l_2^2*(l_1*sin(phi_1) - l_4*sin(phi_4))^2 - ((l_1*sin(phi_1) - l_4*sin(phi_4))^2 + (l_5 - l_1*cos(phi_1) + l_4*cos(phi_4))^2 + l_2^2 - l_3^2)^2 + 4*l_2^2*(l_5 - l_1*cos(phi_1) + l_4*cos(phi_4))^2)^(1/2)) - 2*l_2*l_4*cos(phi_4))/((l_1*sin(phi_1) - l_4*sin(phi_4))^2 + (l_5 - l_1*cos(phi_1) + l_4*cos(phi_4))^2 + l_2^2 - l_3^2 + 2*l_2*(l_5 - l_1*cos(phi_1) + l_4*cos(phi_4))) - (((4*l_2^2*(l_1*sin(phi_1) - l_4*sin(phi_4))^2 - ((l_1*sin(phi_1) - l_4*sin(phi_4))^2 + (l_5 - l_1*cos(phi_1) + l_4*cos(phi_4))^2 + l_2^2 - l_3^2)^2 + 4*l_2^2*(l_5 - l_1*cos(phi_1) + l_4*cos(phi_4))^2)^(1/2) - 2*l_2*(l_1*sin(phi_1) - l_4*sin(phi_4)))*(2*l_2*l_4*sin(phi_4) + 2*l_4*cos(phi_4)*(l_1*sin(phi_1) - l_4*sin(phi_4)) + 2*l_4*sin(phi_4)*(l_5 - l_1*cos(phi_1) + l_4*cos(phi_4))))/((l_1*sin(phi_1) - l_4*sin(phi_4))^2 + (l_5 - l_1*cos(phi_1) + l_4*cos(phi_4))^2 + l_2^2 - l_3^2 + 2*l_2*(l_5 - l_1*cos(phi_1) + l_4*cos(phi_4)))^2)*(l_2*cos(2*atan(((4*l_2^2*(l_1*sin(phi_1) - l_4*sin(phi_4))^2 - ((l_1*sin(phi_1) - l_4*sin(phi_4))^2 + (l_5 - l_1*cos(phi_1) + l_4*cos(phi_4))^2 + l_2^2 - l_3^2)^2 + 4*l_2^2*(l_5 - l_1*cos(phi_1) + l_4*cos(phi_4))^2)^(1/2) - 2*l_2*(l_1*sin(phi_1) - l_4*sin(phi_4)))/((l_1*sin(phi_1) - l_4*sin(phi_4))^2 + (l_5 - l_1*cos(phi_1) + l_4*cos(phi_4))^2 + l_2^2 - l_3^2 + 2*l_2*(l_5 - l_1*cos(phi_1) + l_4*cos(phi_4))))) - l_5/2 + l_1*cos(phi_1)))/(((4*l_2^2*(l_1*sin(phi_1) - l_4*sin(phi_4))^2 - ((l_1*sin(phi_1) - l_4*sin(phi_4))^2 + (l_5 - l_1*cos(phi_1) + l_4*cos(phi_4))^2 + l_2^2 - l_3^2)^2 + 4*l_2^2*(l_5 - l_1*cos(phi_1) + l_4*cos(phi_4))^2)^(1/2) - 2*l_2*(l_1*sin(phi_1) - l_4*sin(phi_4)))^2/((l_1*sin(phi_1) - l_4*sin(phi_4))^2 + (l_5 - l_1*cos(phi_1) + l_4*cos(phi_4))^2 + l_2^2 - l_3^2 + 2*l_2*(l_5 - l_1*cos(phi_1) + l_4*cos(phi_4)))^2 + 1) - (4*l_2*cos(2*atan(((4*l_2^2*(l_1*sin(phi_1) - l_4*sin(phi_4))^2 - ((l_1*sin(phi_1) - l_4*sin(phi_4))^2 + (l_5 - l_1*cos(phi_1) + l_4*cos(phi_4))^2 + l_2^2 - l_3^2)^2 + 4*l_2^2*(l_5 - l_1*cos(phi_1) + l_4*cos(phi_4))^2)^(1/2) - 2*l_2*(l_1*sin(phi_1) - l_4*sin(phi_4)))/((l_1*sin(phi_1) - l_4*sin(phi_4))^2 + (l_5 - l_1*cos(phi_1) + l_4*cos(phi_4))^2 + l_2^2 - l_3^2 + 2*l_2*(l_5 - l_1*cos(phi_1) + l_4*cos(phi_4)))))*(l_2*sin(2*atan(((4*l_2^2*(l_1*sin(phi_1) - l_4*sin(phi_4))^2 - ((l_1*sin(phi_1) - l_4*sin(phi_4))^2 + (l_5 - l_1*cos(phi_1) + l_4*cos(phi_4))^2 + l_2^2 - l_3^2)^2 + 4*l_2^2*(l_5 - l_1*cos(phi_1) + l_4*cos(phi_4))^2)^(1/2) - 2*l_2*(l_1*sin(phi_1) - l_4*sin(phi_4)))/((l_1*sin(phi_1) - l_4*sin(phi_4))^2 + (l_5 - l_1*cos(phi_1) + l_4*cos(phi_4))^2 + l_2^2 - l_3^2 + 2*l_2*(l_5 - l_1*cos(phi_1) + l_4*cos(phi_4))))) + l_1*sin(phi_1))*(((8*l_2^2*l_4*cos(phi_4)*(l_1*sin(phi_1) - l_4*sin(phi_4)) - 2*(2*l_4*cos(phi_4)*(l_1*sin(phi_1) - l_4*sin(phi_4)) + 2*l_4*sin(phi_4)*(l_5 - l_1*cos(phi_1) + l_4*cos(phi_4)))*((l_1*sin(phi_1) - l_4*sin(phi_4))^2 + (l_5 - l_1*cos(phi_1) + l_4*cos(phi_4))^2 + l_2^2 - l_3^2) + 8*l_2^2*l_4*sin(phi_4)*(l_5 - l_1*cos(phi_1) + l_4*cos(phi_4)))/(2*(4*l_2^2*(l_1*sin(phi_1) - l_4*sin(phi_4))^2 - ((l_1*sin(phi_1) - l_4*sin(phi_4))^2 + (l_5 - l_1*cos(phi_1) + l_4*cos(phi_4))^2 + l_2^2 - l_3^2)^2 + 4*l_2^2*(l_5 - l_1*cos(phi_1) + l_4*cos(phi_4))^2)^(1/2)) - 2*l_2*l_4*cos(phi_4))/((l_1*sin(phi_1) - l_4*sin(phi_4))^2 + (l_5 - l_1*cos(phi_1) + l_4*cos(phi_4))^2 + l_2^2 - l_3^2 + 2*l_2*(l_5 - l_1*cos(phi_1) + l_4*cos(phi_4))) - (((4*l_2^2*(l_1*sin(phi_1) - l_4*sin(phi_4))^2 - ((l_1*sin(phi_1) - l_4*sin(phi_4))^2 + (l_5 - l_1*cos(phi_1) + l_4*cos(phi_4))^2 + l_2^2 - l_3^2)^2 + 4*l_2^2*(l_5 - l_1*cos(phi_1) + l_4*cos(phi_4))^2)^(1/2) - 2*l_2*(l_1*sin(phi_1) - l_4*sin(phi_4)))*(2*l_2*l_4*sin(phi_4) + 2*l_4*cos(phi_4)*(l_1*sin(phi_1) - l_4*sin(phi_4)) + 2*l_4*sin(phi_4)*(l_5 - l_1*cos(phi_1) + l_4*cos(phi_4))))/((l_1*sin(phi_1) - l_4*sin(phi_4))^2 + (l_5 - l_1*cos(phi_1) + l_4*cos(phi_4))^2 + l_2^2 - l_3^2 + 2*l_2*(l_5 - l_1*cos(phi_1) + l_4*cos(phi_4)))^2))/(((4*l_2^2*(l_1*sin(phi_1) - l_4*sin(phi_4))^2 - ((l_1*sin(phi_1) - l_4*sin(phi_4))^2 + (l_5 - l_1*cos(phi_1) + l_4*cos(phi_4))^2 + l_2^2 - l_3^2)^2 + 4*l_2^2*(l_5 - l_1*cos(phi_1) + l_4*cos(phi_4))^2)^(1/2) - 2*l_2*(l_1*sin(phi_1) - l_4*sin(phi_4)))^2/((l_1*sin(phi_1) - l_4*sin(phi_4))^2 + (l_5 - l_1*cos(phi_1) + l_4*cos(phi_4))^2 + l_2^2 - l_3^2 + 2*l_2*(l_5 - l_1*cos(phi_1) + l_4*cos(phi_4)))^2 + 1))*(l_2*cos(2*atan(((4*l_2^2*(l_1*sin(phi_1) - l_4*sin(phi_4))^2 - ((l_1*sin(phi_1) - l_4*sin(phi_4))^2 + (l_5 - l_1*cos(phi_1) + l_4*cos(phi_4))^2 + l_2^2 - l_3^2)^2 + 4*l_2^2*(l_5 - l_1*cos(phi_1) + l_4*cos(phi_4))^2)^(1/2) - 2*l_2*(l_1*sin(phi_1) - l_4*sin(phi_4)))/((l_1*sin(phi_1) - l_4*sin(phi_4))^2 + (l_5 - l_1*cos(phi_1) + l_4*cos(phi_4))^2 + l_2^2 - l_3^2 + 2*l_2*(l_5 - l_1*cos(phi_1) + l_4*cos(phi_4))))) - l_5/2 + l_1*cos(phi_1)))/(2*((l_2*sin(2*atan(((4*l_2^2*(l_1*sin(phi_1) - l_4*sin(phi_4))^2 - ((l_1*sin(phi_1) - l_4*sin(phi_4))^2 + (l_5 - l_1*cos(phi_1) + l_4*cos(phi_4))^2 + l_2^2 - l_3^2)^2 + 4*l_2^2*(l_5 - l_1*cos(phi_1) + l_4*cos(phi_4))^2)^(1/2) - 2*l_2*(l_1*sin(phi_1) - l_4*sin(phi_4)))/((l_1*sin(phi_1) - l_4*sin(phi_4))^2 + (l_5 - l_1*cos(phi_1) + l_4*cos(phi_4))^2 + l_2^2 - l_3^2 + 2*l_2*(l_5 - l_1*cos(phi_1) + l_4*cos(phi_4))))) + l_1*sin(phi_1))^2 + (l_2*cos(2*atan(((4*l_2^2*(l_1*sin(phi_1) - l_4*sin(phi_4))^2 - ((l_1*sin(phi_1) - l_4*sin(phi_4))^2 + (l_5 - l_1*cos(phi_1) + l_4*cos(phi_4))^2 + l_2^2 - l_3^2)^2 + 4*l_2^2*(l_5 - l_1*cos(phi_1) + l_4*cos(phi_4))^2)^(1/2) - 2*l_2*(l_1*sin(phi_1) - l_4*sin(phi_4)))/((l_1*sin(phi_1) - l_4*sin(phi_4))^2 + (l_5 - l_1*cos(phi_1) + l_4*cos(phi_4))^2 + l_2^2 - l_3^2 + 2*l_2*(l_5 - l_1*cos(phi_1) + l_4*cos(phi_4))))) - l_5/2 + l_1*cos(phi_1))^2)^(3/2)) - (2*l_2*sin(2*atan(((4*l_2^2*(l_1*sin(phi_1) - l_4*sin(phi_4))^2 - ((l_1*sin(phi_1) - l_4*sin(phi_4))^2 + (l_5 - l_1*cos(phi_1) + l_4*cos(phi_4))^2 + l_2^2 - l_3^2)^2 + 4*l_2^2*(l_5 - l_1*cos(phi_1) + l_4*cos(phi_4))^2)^(1/2) - 2*l_2*(l_1*sin(phi_1) - l_4*sin(phi_4)))/((l_1*sin(phi_1) - l_4*sin(phi_4))^2 + (l_5 - l_1*cos(phi_1) + l_4*cos(phi_4))^2 + l_2^2 - l_3^2 + 2*l_2*(l_5 - l_1*cos(phi_1) + l_4*cos(phi_4)))))*(((8*l_2^2*l_4*cos(phi_4)*(l_1*sin(phi_1) - l_4*sin(phi_4)) - 2*(2*l_4*cos(phi_4)*(l_1*sin(phi_1) - l_4*sin(phi_4)) + 2*l_4*sin(phi_4)*(l_5 - l_1*cos(phi_1) + l_4*cos(phi_4)))*((l_1*sin(phi_1) - l_4*sin(phi_4))^2 + (l_5 - l_1*cos(phi_1) + l_4*cos(phi_4))^2 + l_2^2 - l_3^2) + 8*l_2^2*l_4*sin(phi_4)*(l_5 - l_1*cos(phi_1) + l_4*cos(phi_4)))/(2*(4*l_2^2*(l_1*sin(phi_1) - l_4*sin(phi_4))^2 - ((l_1*sin(phi_1) - l_4*sin(phi_4))^2 + (l_5 - l_1*cos(phi_1) + l_4*cos(phi_4))^2 + l_2^2 - l_3^2)^2 + 4*l_2^2*(l_5 - l_1*cos(phi_1) + l_4*cos(phi_4))^2)^(1/2)) - 2*l_2*l_4*cos(phi_4))/((l_1*sin(phi_1) - l_4*sin(phi_4))^2 + (l_5 - l_1*cos(phi_1) + l_4*cos(phi_4))^2 + l_2^2 - l_3^2 + 2*l_2*(l_5 - l_1*cos(phi_1) + l_4*cos(phi_4))) - (((4*l_2^2*(l_1*sin(phi_1) - l_4*sin(phi_4))^2 - ((l_1*sin(phi_1) - l_4*sin(phi_4))^2 + (l_5 - l_1*cos(phi_1) + l_4*cos(phi_4))^2 + l_2^2 - l_3^2)^2 + 4*l_2^2*(l_5 - l_1*cos(phi_1) + l_4*cos(phi_4))^2)^(1/2) - 2*l_2*(l_1*sin(phi_1) - l_4*sin(phi_4)))*(2*l_2*l_4*sin(phi_4) + 2*l_4*cos(phi_4)*(l_1*sin(phi_1) - l_4*sin(phi_4)) + 2*l_4*sin(phi_4)*(l_5 - l_1*cos(phi_1) + l_4*cos(phi_4))))/((l_1*sin(phi_1) - l_4*sin(phi_4))^2 + (l_5 - l_1*cos(phi_1) + l_4*cos(phi_4))^2 + l_2^2 - l_3^2 + 2*l_2*(l_5 - l_1*cos(phi_1) + l_4*cos(phi_4)))^2))/(((l_2*sin(2*atan(((4*l_2^2*(l_1*sin(phi_1) - l_4*sin(phi_4))^2 - ((l_1*sin(phi_1) - l_4*sin(phi_4))^2 + (l_5 - l_1*cos(phi_1) + l_4*cos(phi_4))^2 + l_2^2 - l_3^2)^2 + 4*l_2^2*(l_5 - l_1*cos(phi_1) + l_4*cos(phi_4))^2)^(1/2) - 2*l_2*(l_1*sin(phi_1) - l_4*sin(phi_4)))/((l_1*sin(phi_1) - l_4*sin(phi_4))^2 + (l_5 - l_1*cos(phi_1) + l_4*cos(phi_4))^2 + l_2^2 - l_3^2 + 2*l_2*(l_5 - l_1*cos(phi_1) + l_4*cos(phi_4))))) + l_1*sin(phi_1))^2 + (l_2*cos(2*atan(((4*l_2^2*(l_1*sin(phi_1) - l_4*sin(phi_4))^2 - ((l_1*sin(phi_1) - l_4*sin(phi_4))^2 + (l_5 - l_1*cos(phi_1) + l_4*cos(phi_4))^2 + l_2^2 - l_3^2)^2 + 4*l_2^2*(l_5 - l_1*cos(phi_1) + l_4*cos(phi_4))^2)^(1/2) - 2*l_2*(l_1*sin(phi_1) - l_4*sin(phi_4)))/((l_1*sin(phi_1) - l_4*sin(phi_4))^2 + (l_5 - l_1*cos(phi_1) + l_4*cos(phi_4))^2 + l_2^2 - l_3^2 + 2*l_2*(l_5 - l_1*cos(phi_1) + l_4*cos(phi_4))))) - l_5/2 + l_1*cos(phi_1))^2)^(1/2)*(((4*l_2^2*(l_1*sin(phi_1) - l_4*sin(phi_4))^2 - ((l_1*sin(phi_1) - l_4*sin(phi_4))^2 + (l_5 - l_1*cos(phi_1) + l_4*cos(phi_4))^2 + l_2^2 - l_3^2)^2 + 4*l_2^2*(l_5 - l_1*cos(phi_1) + l_4*cos(phi_4))^2)^(1/2) - 2*l_2*(l_1*sin(phi_1) - l_4*sin(phi_4)))^2/((l_1*sin(phi_1) - l_4*sin(phi_4))^2 + (l_5 - l_1*cos(phi_1) + l_4*cos(phi_4))^2 + l_2^2 - l_3^2 + 2*l_2*(l_5 - l_1*cos(phi_1) + l_4*cos(phi_4)))^2 + 1)))/(1 - (l_2*cos(2*atan(((4*l_2^2*(l_1*sin(phi_1) - l_4*sin(phi_4))^2 - ((l_1*sin(phi_1) - l_4*sin(phi_4))^2 + (l_5 - l_1*cos(phi_1) + l_4*cos(phi_4))^2 + l_2^2 - l_3^2)^2 + 4*l_2^2*(l_5 - l_1*cos(phi_1) + l_4*cos(phi_4))^2)^(1/2) - 2*l_2*(l_1*sin(phi_1) - l_4*sin(phi_4)))/((l_1*sin(phi_1) - l_4*sin(phi_4))^2 + (l_5 - l_1*cos(phi_1) + l_4*cos(phi_4))^2 + l_2^2 - l_3^2 + 2*l_2*(l_5 - l_1*cos(phi_1) + l_4*cos(phi_4))))) - l_5/2 + l_1*cos(phi_1))^2/((l_2*sin(2*atan(((4*l_2^2*(l_1*sin(phi_1) - l_4*sin(phi_4))^2 - ((l_1*sin(phi_1) - l_4*sin(phi_4))^2 + (l_5 - l_1*cos(phi_1) + l_4*cos(phi_4))^2 + l_2^2 - l_3^2)^2 + 4*l_2^2*(l_5 - l_1*cos(phi_1) + l_4*cos(phi_4))^2)^(1/2) - 2*l_2*(l_1*sin(phi_1) - l_4*sin(phi_4)))/((l_1*sin(phi_1) - l_4*sin(phi_4))^2 + (l_5 - l_1*cos(phi_1) + l_4*cos(phi_4))^2 + l_2^2 - l_3^2 + 2*l_2*(l_5 - l_1*cos(phi_1) + l_4*cos(phi_4))))) + l_1*sin(phi_1))^2 + (l_2*cos(2*atan(((4*l_2^2*(l_1*sin(phi_1) - l_4*sin(phi_4))^2 - ((l_1*sin(phi_1) - l_4*sin(phi_4))^2 + (l_5 - l_1*cos(phi_1) + l_4*cos(phi_4))^2 + l_2^2 - l_3^2)^2 + 4*l_2^2*(l_5 - l_1*cos(phi_1) + l_4*cos(phi_4))^2)^(1/2) - 2*l_2*(l_1*sin(phi_1) - l_4*sin(phi_4)))/((l_1*sin(phi_1) - l_4*sin(phi_4))^2 + (l_5 - l_1*cos(phi_1) + l_4*cos(phi_4))^2 + l_2^2 - l_3^2 + 2*l_2*(l_5 - l_1*cos(phi_1) + l_4*cos(phi_4))))) - l_5/2 + l_1*cos(phi_1))^2))^(1/2);
J_T=[J11,J21;J12,J22];
J_Tinv=inv(J_T);
F=J_Tinv(1,1)*T1+J_Tinv(1,2)*T2;
Tp=J_Tinv(2,1)*T1+J_Tinv(2,2)*T2;
P=F*cos(theta)+Tp*sin(theta)/L_0;
F_N=P+m_w*g+m_w*a_w;

== matlab function Model/右腿LQR/MATLAB Function ==
  data: L_0 input; F_N input; T output; theta input; dtheta input; x input; dx input; phi input; dphi input; Tp output
function [T,Tp]= fcn(L_0,F_N,theta,dtheta,x,dx,phi,dphi)

K11=-172.5944*L_0^3+194.4583*L_0^2-102.6573*L_0-3.2160;
K12=-0.9840*L_0^3+0.4770*L_0^2-8.5684*L_0-0.3764;
K13=-38.8812*L_0^3+40.3986*L_0^2-15.0820*L_0-2.3214;
K14=-25.9829*L_0^3+28.2485*L_0^2-12.5490*L_0-2.7215;
K15=-53.1626*L_0^3+71.4193*L_0^2-37.8708*L_0+9.8810;
K16=-8.7478*L_0^3+11.6234*L_0^2-6.1338*L_0+1.7402;
K21=182.7742*L_0^3-134.1998*L_0^2+17.2318*L_0+11.5442;
K22=5.0007*L_0^3-1.7221*L_0^2-1.6219*L_0+2.0283;
K23=-34.7106*L_0^3+55.1695*L_0^2-32.5200*L_0+8.4420;
K24=-55.6192*L_0^3+72.6502*L_0^2-37.0784*L_0+8.8727;
K25=214.7065*L_0^3-218.2300*L_0^2+79.9589*L_0+4.8045;
K26=36.3354*L_0^3-37.3084*L_0^2+13.9211*L_0+0.5130;

if F_N<20 || F_N>90
    K11=0;
    K12=0;
    K13=0;
    K14=0;
    K15=0;
    K16=0;
    K23=0;
    K24=0;
    K25=0;
    K26=0;
end

T=K11*theta+K12*dtheta+K13*x+K14*dx+K15*phi+K16*dphi;
Tp=K21*theta+K22*dtheta+K23*x+K24*dx+K25*phi+K26*dphi;

== matlab function Model/左腿LQR/MATLAB Function ==
  data: L_0 input; F_N input; T output; theta input; dtheta input; x input; dx input; phi input; dphi input; Tp output
function [T,Tp]= fcn(L_0,F_N,theta,dtheta,x,dx,phi,dphi)

K11=-172.5944*L_0^3+194.4583*L_0^2-102.6573*L_0-3.2160;
K12=-0.9840*L_0^3+0.4770*L_0^2-8.5684*L_0-0.3764;
K13=-38.8812*L_0^3+40.3986*L_0^2-15.0820*L_0-2.3214;
K14=-25.9829*L_0^3+28.2485*L_0^2-12.5490*L_0-2.7215;
K15=-53.1626*L_0^3+71.4193*L_0^2-37.8708*L_0+9.8810;
K16=-8.7478*L_0^3+11.6234*L_0^2-6.1338*L_0+1.7402;
K21=182.7742*L_0^3-134.1998*L_0^2+17.2318*L_0+11.5442;
K22=5.0007*L_0^3-1.7221*L_0^2-1.6219*L_0+2.0283;
K23=-34.7106*L_0^3+55.1695*L_0^2-32.5200*L_0+8.4420;
K24=-55.6192*L_0^3+72.6502*L_0^2-37.0784*L_0+8.8727;
K25=214.7065*L_0^3-218.2300*L_0^2+79.9589*L_0+4.8045;
K26=36.3354*L_0^3-37.3084*L_0^2+13.9211*L_0+0.5130;

if F_N<20 || F_N>90
    K11=0;
    K12=0;
    K13=0;
    K14=0;
    K15=0;
    K16=0;
    K23=0;
    K24=0;
    K25=0;
    K26=0;
end

T=K11*theta+K12*dtheta+K13*x+K14*dx+K15*phi+K16*dphi;
Tp=K21*theta+K22*dtheta+K23*x+K24*dx+K25*phi+K26*dphi;

== matlab function Model/位移补偿/MATLAB Function ==
  data: Target_dx input; Flag output
function Flag = fcn(Target_dx)

Flag=0;
if Target_dx==0
    Flag=1;
end
